simulink model "RFID"  (R2023a)
settings: Solver=VariableStepAuto  StartTime=0.0  StopTime=10.0  RelTol=1e-3
(part 2 of 2)

== system RFID/Profinet_network ==
  Bus Element In2 : Inport  PortName=IOLink_master_Profinet_serial_data_profinet
  Bus Element In1 : Inport  Port=2  PortName="XGSZ84 PNT  _serial_data_Profinet"
  Bus Element In3 : Inport  Port=3  PortName=XGCS 850C 201_Profinet_Data
  Bus Element Out1 : Outport  PortName=Profinet_Sensor_fieldbus

== system RFID/RFID_CANJ ==
  XGCS460B201 : Subsystem
      settings: PortSchema="{\"entries\":[{\"content\":{\"headerSize\":26,\"margin\":15,\"minimumSpacing\":25,\"sides\":[{\"content\":{},\"type\":\"ConnectorPlacement.EquallySpacedRectSide\",\"uuid\":\"ff8f3bf2-d6f6-4ecc-9677-a0e5f5ade440\"},{\"content\":{\"connectorIds\":[\"Out1\"],\"side\":\"RIGHT\"},\"type\":\"ConnectorPlacement.EquallySpacedRectSide\",\"uuid\":\"fe155757-f3d5-40d8-a583-dbbc24843437\"},{\"content\":{\"side\":\"TOP\"},\"type\":\"ConnectorPlacement.EquallySpacedRectSide\",\"uuid\":\"51bc4fd0-0675-45de-93bd-0dc8d94c5489\"}]},\"type\":\"ConnectorPlacement.EquallySpacedConnector\",\"uuid\":\"7eb8fdf8-dbe2-49f3-b9bd-384f85dcc997\"}],\"packageUris\":[\"http://schema.mathworks.com/mf0/Connector/R2020b\"],\"version\":\"1.0\"}"
  XGCS460B202_CANJ_Data1 : Outport  PortName=XGCS460B201_CANJ_Data
  wires:
  XGCS460B201/1(XGCS460B201_CANJ_Data) -> XGCS460B202_CANJ_Data1/1

== system RFID/RFID_EthernetIP ==
  "XGCS 850C 201 " : Subsystem
      settings: PortSchema="{\"entries\":[{\"content\":{\"headerSize\":26,\"margin\":15,\"minimumSpacing\":25,\"sides\":[{\"content\":{},\"type\":\"ConnectorPlacement.EquallySpacedRectSide\",\"uuid\":\"ff8f3bf2-d6f6-4ecc-9677-a0e5f5ade440\"},{\"content\":{\"side\":\"RIGHT\"},\"type\":\"ConnectorPlacement.EquallySpacedRectSide\",\"uuid\":\"fe155757-f3d5-40d8-a583-dbbc24843437\"},{\"content\":{\"connectorIds\":[\"Out1\"],\"side\":\"TOP\"},\"type\":\"ConnectorPlacement.EquallySpacedRectSide\",\"uuid\":\"51bc4fd0-0675-45de-93bd-0dc8d94c5489\"}]},\"type\":\"ConnectorPlacement.EquallySpacedConnector\",\"uuid\":\"7eb8fdf8-dbe2-49f3-b9bd-384f85dcc997\"}],\"packageUris\":[\"http://schema.mathworks.com/mf0/Connector/R2020b\"],\"version\":\"1.0\"}"
  XGCS 850C 201_Ethernetp_Data1 : Outport  PortName=XGCS 850C 201_Ethernetp_Data
  wires:
  "XGCS 850C 201 "/1(XGCS 850C 201_Ethernetp_Data) -> XGCS 850C 201_Ethernetp_Data1/1

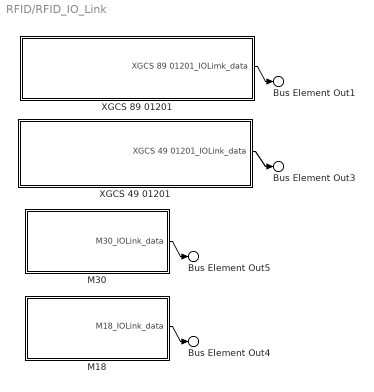
== system RFID/RFID_IO_Link ==
  M18 : Subsystem
      settings: PortSchema="{\"entries\":[{\"content\":{\"headerSize\":26,\"margin\":15,\"minimumSpacing\":25,\"sides\":[{\"content\":{},\"type\":\"ConnectorPlacement.EquallySpacedRectSide\",\"uuid\":\"ff8f3bf2-d6f6-4ecc-9677-a0e5f5ade440\"},{\"content\":{\"connectorIds\":[\"Out1\"],\"side\":\"RIGHT\"},\"type\":\"ConnectorPlacement.EquallySpacedRectSide\",\"uuid\":\"fe155757-f3d5-40d8-a583-dbbc24843437\"},{\"content\":{\"side\":\"TOP\"},\"type\":\"ConnectorPlacement.EquallySpacedRectSide\",\"uuid\":\"51bc4fd0-0675-45de-93bd-0dc8d94c5489\"}]},\"type\":\"ConnectorPlacement.EquallySpacedConnector\",\"uuid\":\"7eb8fdf8-dbe2-49f3-b9bd-384f85dcc997\"}],\"packageUris\":[\"http://schema.mathworks.com/mf0/Connector/R2020b\"],\"version\":\"1.0\"}"
  M30 : Subsystem
      settings: PortSchema="{\"entries\":[{\"content\":{\"headerSize\":26,\"margin\":15,\"minimumSpacing\":25,\"sides\":[{\"content\":{},\"type\":\"ConnectorPlacement.EquallySpacedRectSide\",\"uuid\":\"ff8f3bf2-d6f6-4ecc-9677-a0e5f5ade440\"},{\"content\":{\"connectorIds\":[\"Out1\"],\"side\":\"RIGHT\"},\"type\":\"ConnectorPlacement.EquallySpacedRectSide\",\"uuid\":\"fe155757-f3d5-40d8-a583-dbbc24843437\"},{\"content\":{\"side\":\"TOP\"},\"type\":\"ConnectorPlacement.EquallySpacedRectSide\",\"uuid\":\"51bc4fd0-0675-45de-93bd-0dc8d94c5489\"}]},\"type\":\"ConnectorPlacement.EquallySpacedConnector\",\"uuid\":\"7eb8fdf8-dbe2-49f3-b9bd-384f85dcc997\"}],\"packageUris\":[\"http://schema.mathworks.com/mf0/Connector/R2020b\"],\"version\":\"1.0\"}"
  XGCS 49 01201 : Subsystem
      settings: PortSchema="{\"entries\":[{\"content\":{\"headerSize\":26,\"margin\":15,\"minimumSpacing\":25,\"sides\":[{\"content\":{},\"type\":\"ConnectorPlacement.EquallySpacedRectSide\",\"uuid\":\"ff8f3bf2-d6f6-4ecc-9677-a0e5f5ade440\"},{\"content\":{\"connectorIds\":[\"Out1\"],\"side\":\"RIGHT\"},\"type\":\"ConnectorPlacement.EquallySpacedRectSide\",\"uuid\":\"fe155757-f3d5-40d8-a583-dbbc24843437\"},{\"content\":{\"side\":\"TOP\"},\"type\":\"ConnectorPlacement.EquallySpacedRectSide\",\"uuid\":\"51bc4fd0-0675-45de-93bd-0dc8d94c5489\"}]},\"type\":\"ConnectorPlacement.EquallySpacedConnector\",\"uuid\":\"7eb8fdf8-dbe2-49f3-b9bd-384f85dcc997\"}],\"packageUris\":[\"http://schema.mathworks.com/mf0/Connector/R2020b\"],\"version\":\"1.0\"}"
  XGCS 89 01201 : Subsystem
      settings: PortSchema="{\"entries\":[{\"content\":{\"headerSize\":26,\"margin\":15,\"minimumSpacing\":25,\"sides\":[{\"content\":{},\"type\":\"ConnectorPlacement.EquallySpacedRectSide\",\"uuid\":\"ff8f3bf2-d6f6-4ecc-9677-a0e5f5ade440\"},{\"content\":{\"connectorIds\":[\"Out1\"],\"side\":\"RIGHT\"},\"type\":\"ConnectorPlacement.EquallySpacedRectSide\",\"uuid\":\"fe155757-f3d5-40d8-a583-dbbc24843437\"},{\"content\":{\"side\":\"TOP\"},\"type\":\"ConnectorPlacement.EquallySpacedRectSide\",\"uuid\":\"51bc4fd0-0675-45de-93bd-0dc8d94c5489\"}]},\"type\":\"ConnectorPlacement.EquallySpacedConnector\",\"uuid\":\"7eb8fdf8-dbe2-49f3-b9bd-384f85dcc997\"}],\"packageUris\":[\"http://schema.mathworks.com/mf0/Connector/R2020b\"],\"version\":\"1.0\"}"
  Bus Element Out1 : Outport  PortName=XGCS 89 01201_IOLimk_data
  Bus Element Out3 : Outport  Port=2  PortName=XGCS 49 01201_IOLink_data
  Bus Element Out4 : Outport  Port=3  PortName=M18_IOLink_data
  Bus Element Out5 : Outport  Port=4  PortName=M30_IOLink_data
  wires:
  XGCS 89 01201/1(XGCS 89 01201_IOLimk_data) -> Bus Element Out1/1
  XGCS 49 01201/1(XGCS 49 01201_IOLink_data) -> Bus Element Out3/1
  M30/1(M30_IOLink_data) -> Bus Element Out5/1
  M18/1(M18_IOLink_data) -> Bus Element Out4/1

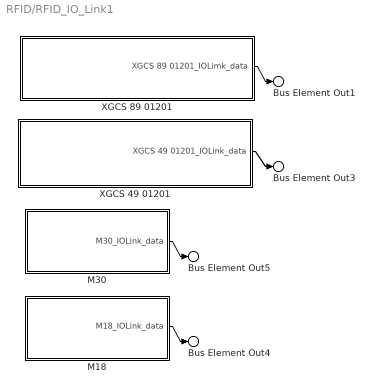
== system RFID/RFID_IO_Link1 ==
  M18 : Subsystem
      settings: PortSchema="{\"entries\":[{\"content\":{\"headerSize\":26,\"margin\":15,\"minimumSpacing\":25,\"sides\":[{\"content\":{},\"type\":\"ConnectorPlacement.EquallySpacedRectSide\",\"uuid\":\"ff8f3bf2-d6f6-4ecc-9677-a0e5f5ade440\"},{\"content\":{\"connectorIds\":[\"Out1\"],\"side\":\"RIGHT\"},\"type\":\"ConnectorPlacement.EquallySpacedRectSide\",\"uuid\":\"fe155757-f3d5-40d8-a583-dbbc24843437\"},{\"content\":{\"side\":\"TOP\"},\"type\":\"ConnectorPlacement.EquallySpacedRectSide\",\"uuid\":\"51bc4fd0-0675-45de-93bd-0dc8d94c5489\"}]},\"type\":\"ConnectorPlacement.EquallySpacedConnector\",\"uuid\":\"7eb8fdf8-dbe2-49f3-b9bd-384f85dcc997\"}],\"packageUris\":[\"http://schema.mathworks.com/mf0/Connector/R2020b\"],\"version\":\"1.0\"}"
  M30 : Subsystem
      settings: PortSchema="{\"entries\":[{\"content\":{\"headerSize\":26,\"margin\":15,\"minimumSpacing\":25,\"sides\":[{\"content\":{},\"type\":\"ConnectorPlacement.EquallySpacedRectSide\",\"uuid\":\"ff8f3bf2-d6f6-4ecc-9677-a0e5f5ade440\"},{\"content\":{\"connectorIds\":[\"Out1\"],\"side\":\"RIGHT\"},\"type\":\"ConnectorPlacement.EquallySpacedRectSide\",\"uuid\":\"fe155757-f3d5-40d8-a583-dbbc24843437\"},{\"content\":{\"side\":\"TOP\"},\"type\":\"ConnectorPlacement.EquallySpacedRectSide\",\"uuid\":\"51bc4fd0-0675-45de-93bd-0dc8d94c5489\"}]},\"type\":\"ConnectorPlacement.EquallySpacedConnector\",\"uuid\":\"7eb8fdf8-dbe2-49f3-b9bd-384f85dcc997\"}],\"packageUris\":[\"http://schema.mathworks.com/mf0/Connector/R2020b\"],\"version\":\"1.0\"}"
  XGCS 49 01201 : Subsystem
      settings: PortSchema="{\"entries\":[{\"content\":{\"headerSize\":26,\"margin\":15,\"minimumSpacing\":25,\"sides\":[{\"content\":{},\"type\":\"ConnectorPlacement.EquallySpacedRectSide\",\"uuid\":\"ff8f3bf2-d6f6-4ecc-9677-a0e5f5ade440\"},{\"content\":{\"connectorIds\":[\"Out1\"],\"side\":\"RIGHT\"},\"type\":\"ConnectorPlacement.EquallySpacedRectSide\",\"uuid\":\"fe155757-f3d5-40d8-a583-dbbc24843437\"},{\"content\":{\"side\":\"TOP\"},\"type\":\"ConnectorPlacement.EquallySpacedRectSide\",\"uuid\":\"51bc4fd0-0675-45de-93bd-0dc8d94c5489\"}]},\"type\":\"ConnectorPlacement.EquallySpacedConnector\",\"uuid\":\"7eb8fdf8-dbe2-49f3-b9bd-384f85dcc997\"}],\"packageUris\":[\"http://schema.mathworks.com/mf0/Connector/R2020b\"],\"version\":\"1.0\"}"
  XGCS 89 01201 : Subsystem
      settings: PortSchema="{\"entries\":[{\"content\":{\"headerSize\":26,\"margin\":15,\"minimumSpacing\":25,\"sides\":[{\"content\":{},\"type\":\"ConnectorPlacement.EquallySpacedRectSide\",\"uuid\":\"ff8f3bf2-d6f6-4ecc-9677-a0e5f5ade440\"},{\"content\":{\"connectorIds\":[\"Out1\"],\"side\":\"RIGHT\"},\"type\":\"ConnectorPlacement.EquallySpacedRectSide\",\"uuid\":\"fe155757-f3d5-40d8-a583-dbbc24843437\"},{\"content\":{\"side\":\"TOP\"},\"type\":\"ConnectorPlacement.EquallySpacedRectSide\",\"uuid\":\"51bc4fd0-0675-45de-93bd-0dc8d94c5489\"}]},\"type\":\"ConnectorPlacement.EquallySpacedConnector\",\"uuid\":\"7eb8fdf8-dbe2-49f3-b9bd-384f85dcc997\"}],\"packageUris\":[\"http://schema.mathworks.com/mf0/Connector/R2020b\"],\"version\":\"1.0\"}"
  Bus Element Out1 : Outport  PortName=XGCS 89 01201_IOLimk_data
  Bus Element Out3 : Outport  Port=2  PortName=XGCS 49 01201_IOLink_data
  Bus Element Out4 : Outport  Port=3  PortName=M18_IOLink_data
  Bus Element Out5 : Outport  Port=4  PortName=M30_IOLink_data
  wires:
  XGCS 89 01201/1(XGCS 89 01201_IOLimk_data) -> Bus Element Out1/1
  XGCS 49 01201/1(XGCS 49 01201_IOLink_data) -> Bus Element Out3/1
  M30/1(M30_IOLink_data) -> Bus Element Out5/1
  M18/1(M18_IOLink_data) -> Bus Element Out4/1

== system RFID/RFID_Modbus ==
  XGCS 850C 201 : Subsystem
      settings: PortSchema="{\"entries\":[{\"content\":{\"headerSize\":26,\"margin\":15,\"minimumSpacing\":25,\"sides\":[{\"content\":{},\"type\":\"ConnectorPlacement.EquallySpacedRectSide\",\"uuid\":\"ff8f3bf2-d6f6-4ecc-9677-a0e5f5ade440\"},{\"content\":{\"side\":\"RIGHT\"},\"type\":\"ConnectorPlacement.EquallySpacedRectSide\",\"uuid\":\"fe155757-f3d5-40d8-a583-dbbc24843437\"},{\"content\":{\"connectorIds\":[\"Out1\"],\"side\":\"TOP\"},\"type\":\"ConnectorPlacement.EquallySpacedRectSide\",\"uuid\":\"51bc4fd0-0675-45de-93bd-0dc8d94c5489\"}]},\"type\":\"ConnectorPlacement.EquallySpacedConnector\",\"uuid\":\"7eb8fdf8-dbe2-49f3-b9bd-384f85dcc997\"}],\"packageUris\":[\"http://schema.mathworks.com/mf0/Connector/R2020b\"],\"version\":\"1.0\"}"
  XGCS 850C 201_ModusTCp_Data1 : Outport  PortName=XGCS 850C 201_ModusTCp_Data
  wires:
  XGCS 850C 201/1(XGCS 850C 201_ModusTCp_Data) -> XGCS 850C 201_ModusTCp_Data1/1

== system RFID/RFID_PNP ==
  "XGCS49 1 B201 " : Subsystem
      settings: PortSchema="{\"entries\":[{\"content\":{\"headerSize\":26,\"margin\":15,\"minimumSpacing\":25,\"sides\":[{\"content\":{},\"type\":\"ConnectorPlacement.EquallySpacedRectSide\",\"uuid\":\"ff8f3bf2-d6f6-4ecc-9677-a0e5f5ade440\"},{\"content\":{\"connectorIds\":[\"Out1\"],\"side\":\"RIGHT\"},\"type\":\"ConnectorPlacement.EquallySpacedRectSide\",\"uuid\":\"fe155757-f3d5-40d8-a583-dbbc24843437\"},{\"content\":{\"side\":\"TOP\"},\"type\":\"ConnectorPlacement.EquallySpacedRectSide\",\"uuid\":\"51bc4fd0-0675-45de-93bd-0dc8d94c5489\"}]},\"type\":\"ConnectorPlacement.EquallySpacedConnector\",\"uuid\":\"7eb8fdf8-dbe2-49f3-b9bd-384f85dcc997\"}],\"packageUris\":[\"http://schema.mathworks.com/mf0/Connector/R2020b\"],\"version\":\"1.0\"}"
  XGCS49 1 B201_PNP_Data1 : Outport  PortName=XGCS49 1 B201_PNP_Data
  wires:
  "XGCS49 1 B201 "/1(XGCS49 1 B201_PNP_Data) -> XGCS49 1 B201_PNP_Data1/1

== system RFID/RFID_Profinet ==
  "XGCS 850C 201 " : Subsystem
      settings: PortSchema="{\"entries\":[{\"content\":{\"headerSize\":26,\"margin\":15,\"minimumSpacing\":25,\"sides\":[{\"content\":{},\"type\":\"ConnectorPlacement.EquallySpacedRectSide\",\"uuid\":\"ff8f3bf2-d6f6-4ecc-9677-a0e5f5ade440\"},{\"content\":{\"side\":\"RIGHT\"},\"type\":\"ConnectorPlacement.EquallySpacedRectSide\",\"uuid\":\"fe155757-f3d5-40d8-a583-dbbc24843437\"},{\"content\":{\"connectorIds\":[\"Out1\"],\"side\":\"TOP\"},\"type\":\"ConnectorPlacement.EquallySpacedRectSide\",\"uuid\":\"51bc4fd0-0675-45de-93bd-0dc8d94c5489\"}]},\"type\":\"ConnectorPlacement.EquallySpacedConnector\",\"uuid\":\"7eb8fdf8-dbe2-49f3-b9bd-384f85dcc997\"}],\"packageUris\":[\"http://schema.mathworks.com/mf0/Connector/R2020b\"],\"version\":\"1.0\"}"
  Bus Element Out1 : Outport  PortName=XGCS 850C 201_Profinet_Data
  wires:
  "XGCS 850C 201 "/1(XGCS 850C 201_Profinet_Data) -> Bus Element Out1/1

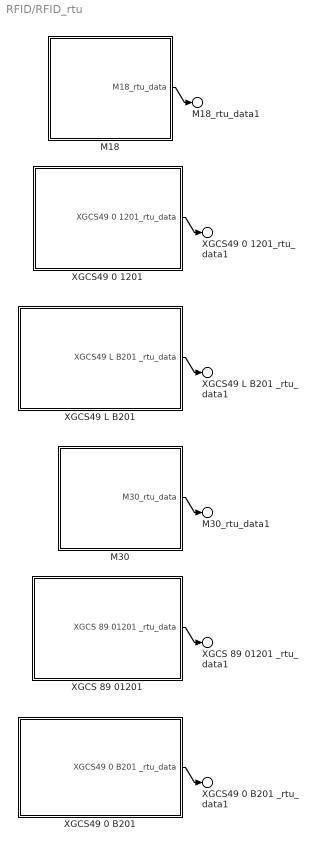
== system RFID/RFID_rtu ==
  M18 : Subsystem
      settings: PortSchema="{\"entries\":[{\"content\":{\"headerSize\":26,\"margin\":15,\"minimumSpacing\":25,\"sides\":[{\"content\":{},\"type\":\"ConnectorPlacement.EquallySpacedRectSide\",\"uuid\":\"ff8f3bf2-d6f6-4ecc-9677-a0e5f5ade440\"},{\"content\":{\"connectorIds\":[\"Out1\"],\"side\":\"RIGHT\"},\"type\":\"ConnectorPlacement.EquallySpacedRectSide\",\"uuid\":\"fe155757-f3d5-40d8-a583-dbbc24843437\"},{\"content\":{\"side\":\"TOP\"},\"type\":\"ConnectorPlacement.EquallySpacedRectSide\",\"uuid\":\"51bc4fd0-0675-45de-93bd-0dc8d94c5489\"}]},\"type\":\"ConnectorPlacement.EquallySpacedConnector\",\"uuid\":\"7eb8fdf8-dbe2-49f3-b9bd-384f85dcc997\"}],\"packageUris\":[\"http://schema.mathworks.com/mf0/Connector/R2020b\"],\"version\":\"1.0\"}"
  M30 : Subsystem
      settings: PortSchema="{\"entries\":[{\"content\":{\"headerSize\":26,\"margin\":15,\"minimumSpacing\":25,\"sides\":[{\"content\":{},\"type\":\"ConnectorPlacement.EquallySpacedRectSide\",\"uuid\":\"ff8f3bf2-d6f6-4ecc-9677-a0e5f5ade440\"},{\"content\":{\"connectorIds\":[\"Out1\"],\"side\":\"RIGHT\"},\"type\":\"ConnectorPlacement.EquallySpacedRectSide\",\"uuid\":\"fe155757-f3d5-40d8-a583-dbbc24843437\"},{\"content\":{\"side\":\"TOP\"},\"type\":\"ConnectorPlacement.EquallySpacedRectSide\",\"uuid\":\"51bc4fd0-0675-45de-93bd-0dc8d94c5489\"}]},\"type\":\"ConnectorPlacement.EquallySpacedConnector\",\"uuid\":\"7eb8fdf8-dbe2-49f3-b9bd-384f85dcc997\"}],\"packageUris\":[\"http://schema.mathworks.com/mf0/Connector/R2020b\"],\"version\":\"1.0\"}"
  "XGCS 89 01201 " : Subsystem
      settings: PortSchema="{\"entries\":[{\"content\":{\"headerSize\":26,\"margin\":15,\"minimumSpacing\":25,\"sides\":[{\"content\":{},\"type\":\"ConnectorPlacement.EquallySpacedRectSide\",\"uuid\":\"ff8f3bf2-d6f6-4ecc-9677-a0e5f5ade440\"},{\"content\":{\"connectorIds\":[\"Out1\"],\"side\":\"RIGHT\"},\"type\":\"ConnectorPlacement.EquallySpacedRectSide\",\"uuid\":\"fe155757-f3d5-40d8-a583-dbbc24843437\"},{\"content\":{\"side\":\"TOP\"},\"type\":\"ConnectorPlacement.EquallySpacedRectSide\",\"uuid\":\"51bc4fd0-0675-45de-93bd-0dc8d94c5489\"}]},\"type\":\"ConnectorPlacement.EquallySpacedConnector\",\"uuid\":\"7eb8fdf8-dbe2-49f3-b9bd-384f85dcc997\"}],\"packageUris\":[\"http://schema.mathworks.com/mf0/Connector/R2020b\"],\"version\":\"1.0\"}"
  "XGCS49 0 1201 " : Subsystem
      settings: PortSchema="{\"entries\":[{\"content\":{\"headerSize\":26,\"margin\":15,\"minimumSpacing\":25,\"sides\":[{\"content\":{},\"type\":\"ConnectorPlacement.EquallySpacedRectSide\",\"uuid\":\"ff8f3bf2-d6f6-4ecc-9677-a0e5f5ade440\"},{\"content\":{\"connectorIds\":[\"Out1\"],\"side\":\"RIGHT\"},\"type\":\"ConnectorPlacement.EquallySpacedRectSide\",\"uuid\":\"fe155757-f3d5-40d8-a583-dbbc24843437\"},{\"content\":{\"side\":\"TOP\"},\"type\":\"ConnectorPlacement.EquallySpacedRectSide\",\"uuid\":\"51bc4fd0-0675-45de-93bd-0dc8d94c5489\"}]},\"type\":\"ConnectorPlacement.EquallySpacedConnector\",\"uuid\":\"7eb8fdf8-dbe2-49f3-b9bd-384f85dcc997\"}],\"packageUris\":[\"http://schema.mathworks.com/mf0/Connector/R2020b\"],\"version\":\"1.0\"}"
  "XGCS49 0 B201 " : Subsystem
      settings: PortSchema="{\"entries\":[{\"content\":{\"headerSize\":26,\"margin\":15,\"minimumSpacing\":25,\"sides\":[{\"content\":{},\"type\":\"ConnectorPlacement.EquallySpacedRectSide\",\"uuid\":\"ff8f3bf2-d6f6-4ecc-9677-a0e5f5ade440\"},{\"content\":{\"connectorIds\":[\"Out1\"],\"side\":\"RIGHT\"},\"type\":\"ConnectorPlacement.EquallySpacedRectSide\",\"uuid\":\"fe155757-f3d5-40d8-a583-dbbc24843437\"},{\"content\":{\"side\":\"TOP\"},\"type\":\"ConnectorPlacement.EquallySpacedRectSide\",\"uuid\":\"51bc4fd0-0675-45de-93bd-0dc8d94c5489\"}]},\"type\":\"ConnectorPlacement.EquallySpacedConnector\",\"uuid\":\"7eb8fdf8-dbe2-49f3-b9bd-384f85dcc997\"}],\"packageUris\":[\"http://schema.mathworks.com/mf0/Connector/R2020b\"],\"version\":\"1.0\"}"
  "XGCS49 L B201 " : Subsystem
      settings: PortSchema="{\"entries\":[{\"content\":{\"headerSize\":26,\"margin\":15,\"minimumSpacing\":25,\"sides\":[{\"content\":{},\"type\":\"ConnectorPlacement.EquallySpacedRectSide\",\"uuid\":\"ff8f3bf2-d6f6-4ecc-9677-a0e5f5ade440\"},{\"content\":{\"connectorIds\":[\"Out1\"],\"side\":\"RIGHT\"},\"type\":\"ConnectorPlacement.EquallySpacedRectSide\",\"uuid\":\"fe155757-f3d5-40d8-a583-dbbc24843437\"},{\"content\":{\"side\":\"TOP\"},\"type\":\"ConnectorPlacement.EquallySpacedRectSide\",\"uuid\":\"51bc4fd0-0675-45de-93bd-0dc8d94c5489\"}]},\"type\":\"ConnectorPlacement.EquallySpacedConnector\",\"uuid\":\"7eb8fdf8-dbe2-49f3-b9bd-384f85dcc997\"}],\"packageUris\":[\"http://schema.mathworks.com/mf0/Connector/R2020b\"],\"version\":\"1.0\"}"
  M18_rtu_data1 : Outport  PortName=M18_rtu_data
  M30_rtu_data1 : Outport  Port=2  PortName=M30_rtu_data
  XGCS49 0 1201_rtu_data1 : Outport  Port=3  PortName=XGCS49 0 1201_rtu_data
  XGCS 89 01201 _rtu_data1 : Outport  Port=4  PortName=XGCS 89 01201 _rtu_data
  XGCS49 0 B201 _rtu_data1 : Outport  Port=5  PortName=XGCS49 0 B201 _rtu_data
  XGCS49 L B201 _rtu_data1 : Outport  Port=6  PortName=XGCS49 L B201 _rtu_data
  wires:
  "XGCS 89 01201 "/1(XGCS 89 01201 _rtu_data) -> XGCS 89 01201 _rtu_data1/1
  "XGCS49 L B201 "/1(XGCS49 L B201 _rtu_data) -> XGCS49 L B201 _rtu_data1/1
  "XGCS49 0 B201 "/1(XGCS49 0 B201 _rtu_data) -> XGCS49 0 B201 _rtu_data1/1
  M18/1(M18_rtu_data) -> M18_rtu_data1/1
  M30/1(M30_rtu_data) -> M30_rtu_data1/1
  "XGCS49 0 1201 "/1(XGCS49 0 1201_rtu_data) -> XGCS49 0 1201_rtu_data1/1

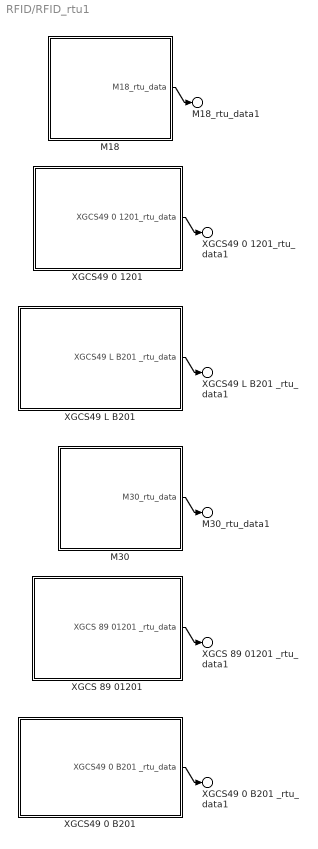
== system RFID/RFID_rtu1 ==
  M18 : Subsystem
      settings: PortSchema="{\"entries\":[{\"content\":{\"headerSize\":26,\"margin\":15,\"minimumSpacing\":25,\"sides\":[{\"content\":{},\"type\":\"ConnectorPlacement.EquallySpacedRectSide\",\"uuid\":\"ff8f3bf2-d6f6-4ecc-9677-a0e5f5ade440\"},{\"content\":{\"connectorIds\":[\"Out1\"],\"side\":\"RIGHT\"},\"type\":\"ConnectorPlacement.EquallySpacedRectSide\",\"uuid\":\"fe155757-f3d5-40d8-a583-dbbc24843437\"},{\"content\":{\"side\":\"TOP\"},\"type\":\"ConnectorPlacement.EquallySpacedRectSide\",\"uuid\":\"51bc4fd0-0675-45de-93bd-0dc8d94c5489\"}]},\"type\":\"ConnectorPlacement.EquallySpacedConnector\",\"uuid\":\"7eb8fdf8-dbe2-49f3-b9bd-384f85dcc997\"}],\"packageUris\":[\"http://schema.mathworks.com/mf0/Connector/R2020b\"],\"version\":\"1.0\"}"
  M30 : Subsystem
      settings: PortSchema="{\"entries\":[{\"content\":{\"headerSize\":26,\"margin\":15,\"minimumSpacing\":25,\"sides\":[{\"content\":{},\"type\":\"ConnectorPlacement.EquallySpacedRectSide\",\"uuid\":\"ff8f3bf2-d6f6-4ecc-9677-a0e5f5ade440\"},{\"content\":{\"connectorIds\":[\"Out1\"],\"side\":\"RIGHT\"},\"type\":\"ConnectorPlacement.EquallySpacedRectSide\",\"uuid\":\"fe155757-f3d5-40d8-a583-dbbc24843437\"},{\"content\":{\"side\":\"TOP\"},\"type\":\"ConnectorPlacement.EquallySpacedRectSide\",\"uuid\":\"51bc4fd0-0675-45de-93bd-0dc8d94c5489\"}]},\"type\":\"ConnectorPlacement.EquallySpacedConnector\",\"uuid\":\"7eb8fdf8-dbe2-49f3-b9bd-384f85dcc997\"}],\"packageUris\":[\"http://schema.mathworks.com/mf0/Connector/R2020b\"],\"version\":\"1.0\"}"
  "XGCS 89 01201 " : Subsystem
      settings: PortSchema="{\"entries\":[{\"content\":{\"headerSize\":26,\"margin\":15,\"minimumSpacing\":25,\"sides\":[{\"content\":{},\"type\":\"ConnectorPlacement.EquallySpacedRectSide\",\"uuid\":\"ff8f3bf2-d6f6-4ecc-9677-a0e5f5ade440\"},{\"content\":{\"connectorIds\":[\"Out1\"],\"side\":\"RIGHT\"},\"type\":\"ConnectorPlacement.EquallySpacedRectSide\",\"uuid\":\"fe155757-f3d5-40d8-a583-dbbc24843437\"},{\"content\":{\"side\":\"TOP\"},\"type\":\"ConnectorPlacement.EquallySpacedRectSide\",\"uuid\":\"51bc4fd0-0675-45de-93bd-0dc8d94c5489\"}]},\"type\":\"ConnectorPlacement.EquallySpacedConnector\",\"uuid\":\"7eb8fdf8-dbe2-49f3-b9bd-384f85dcc997\"}],\"packageUris\":[\"http://schema.mathworks.com/mf0/Connector/R2020b\"],\"version\":\"1.0\"}"
  "XGCS49 0 1201 " : Subsystem
      settings: PortSchema="{\"entries\":[{\"content\":{\"headerSize\":26,\"margin\":15,\"minimumSpacing\":25,\"sides\":[{\"content\":{},\"type\":\"ConnectorPlacement.EquallySpacedRectSide\",\"uuid\":\"ff8f3bf2-d6f6-4ecc-9677-a0e5f5ade440\"},{\"content\":{\"connectorIds\":[\"Out1\"],\"side\":\"RIGHT\"},\"type\":\"ConnectorPlacement.EquallySpacedRectSide\",\"uuid\":\"fe155757-f3d5-40d8-a583-dbbc24843437\"},{\"content\":{\"side\":\"TOP\"},\"type\":\"ConnectorPlacement.EquallySpacedRectSide\",\"uuid\":\"51bc4fd0-0675-45de-93bd-0dc8d94c5489\"}]},\"type\":\"ConnectorPlacement.EquallySpacedConnector\",\"uuid\":\"7eb8fdf8-dbe2-49f3-b9bd-384f85dcc997\"}],\"packageUris\":[\"http://schema.mathworks.com/mf0/Connector/R2020b\"],\"version\":\"1.0\"}"
  "XGCS49 0 B201 " : Subsystem
      settings: PortSchema="{\"entries\":[{\"content\":{\"headerSize\":26,\"margin\":15,\"minimumSpacing\":25,\"sides\":[{\"content\":{},\"type\":\"ConnectorPlacement.EquallySpacedRectSide\",\"uuid\":\"ff8f3bf2-d6f6-4ecc-9677-a0e5f5ade440\"},{\"content\":{\"connectorIds\":[\"Out1\"],\"side\":\"RIGHT\"},\"type\":\"ConnectorPlacement.EquallySpacedRectSide\",\"uuid\":\"fe155757-f3d5-40d8-a583-dbbc24843437\"},{\"content\":{\"side\":\"TOP\"},\"type\":\"ConnectorPlacement.EquallySpacedRectSide\",\"uuid\":\"51bc4fd0-0675-45de-93bd-0dc8d94c5489\"}]},\"type\":\"ConnectorPlacement.EquallySpacedConnector\",\"uuid\":\"7eb8fdf8-dbe2-49f3-b9bd-384f85dcc997\"}],\"packageUris\":[\"http://schema.mathworks.com/mf0/Connector/R2020b\"],\"version\":\"1.0\"}"
  "XGCS49 L B201 " : Subsystem
      settings: PortSchema="{\"entries\":[{\"content\":{\"headerSize\":26,\"margin\":15,\"minimumSpacing\":25,\"sides\":[{\"content\":{},\"type\":\"ConnectorPlacement.EquallySpacedRectSide\",\"uuid\":\"ff8f3bf2-d6f6-4ecc-9677-a0e5f5ade440\"},{\"content\":{\"connectorIds\":[\"Out1\"],\"side\":\"RIGHT\"},\"type\":\"ConnectorPlacement.EquallySpacedRectSide\",\"uuid\":\"fe155757-f3d5-40d8-a583-dbbc24843437\"},{\"content\":{\"side\":\"TOP\"},\"type\":\"ConnectorPlacement.EquallySpacedRectSide\",\"uuid\":\"51bc4fd0-0675-45de-93bd-0dc8d94c5489\"}]},\"type\":\"ConnectorPlacement.EquallySpacedConnector\",\"uuid\":\"7eb8fdf8-dbe2-49f3-b9bd-384f85dcc997\"}],\"packageUris\":[\"http://schema.mathworks.com/mf0/Connector/R2020b\"],\"version\":\"1.0\"}"
  M18_rtu_data1 : Outport  PortName=M18_rtu_data
  M30_rtu_data1 : Outport  Port=2  PortName=M30_rtu_data
  XGCS49 0 1201_rtu_data1 : Outport  Port=3  PortName=XGCS49 0 1201_rtu_data
  XGCS 89 01201 _rtu_data1 : Outport  Port=4  PortName=XGCS 89 01201 _rtu_data
  XGCS49 0 B201 _rtu_data1 : Outport  Port=5  PortName=XGCS49 0 B201 _rtu_data
  XGCS49 L B201 _rtu_data1 : Outport  Port=6  PortName=XGCS49 L B201 _rtu_data
  wires:
  "XGCS 89 01201 "/1(XGCS 89 01201 _rtu_data) -> XGCS 89 01201 _rtu_data1/1
  "XGCS49 L B201 "/1(XGCS49 L B201 _rtu_data) -> XGCS49 L B201 _rtu_data1/1
  "XGCS49 0 B201 "/1(XGCS49 0 B201 _rtu_data) -> XGCS49 0 B201 _rtu_data1/1
  M18/1(M18_rtu_data) -> M18_rtu_data1/1
  M30/1(M30_rtu_data) -> M30_rtu_data1/1
  "XGCS49 0 1201 "/1(XGCS49 0 1201_rtu_data) -> XGCS49 0 1201_rtu_data1/1

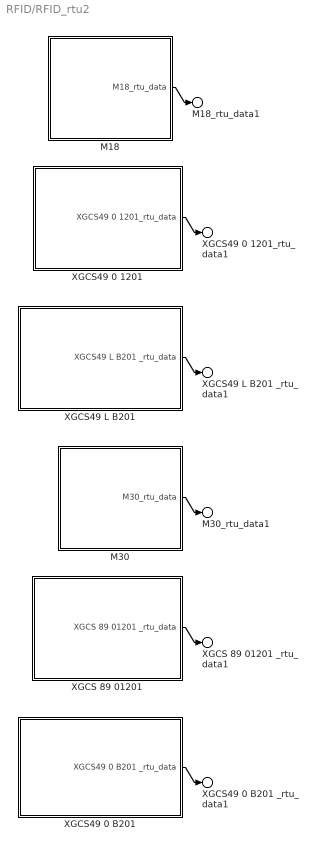
== system RFID/RFID_rtu2 ==
  M18 : Subsystem
      settings: PortSchema="{\"entries\":[{\"content\":{\"headerSize\":26,\"margin\":15,\"minimumSpacing\":25,\"sides\":[{\"content\":{},\"type\":\"ConnectorPlacement.EquallySpacedRectSide\",\"uuid\":\"ff8f3bf2-d6f6-4ecc-9677-a0e5f5ade440\"},{\"content\":{\"connectorIds\":[\"Out1\"],\"side\":\"RIGHT\"},\"type\":\"ConnectorPlacement.EquallySpacedRectSide\",\"uuid\":\"fe155757-f3d5-40d8-a583-dbbc24843437\"},{\"content\":{\"side\":\"TOP\"},\"type\":\"ConnectorPlacement.EquallySpacedRectSide\",\"uuid\":\"51bc4fd0-0675-45de-93bd-0dc8d94c5489\"}]},\"type\":\"ConnectorPlacement.EquallySpacedConnector\",\"uuid\":\"7eb8fdf8-dbe2-49f3-b9bd-384f85dcc997\"}],\"packageUris\":[\"http://schema.mathworks.com/mf0/Connector/R2020b\"],\"version\":\"1.0\"}"
  M30 : Subsystem
      settings: PortSchema="{\"entries\":[{\"content\":{\"headerSize\":26,\"margin\":15,\"minimumSpacing\":25,\"sides\":[{\"content\":{},\"type\":\"ConnectorPlacement.EquallySpacedRectSide\",\"uuid\":\"ff8f3bf2-d6f6-4ecc-9677-a0e5f5ade440\"},{\"content\":{\"connectorIds\":[\"Out1\"],\"side\":\"RIGHT\"},\"type\":\"ConnectorPlacement.EquallySpacedRectSide\",\"uuid\":\"fe155757-f3d5-40d8-a583-dbbc24843437\"},{\"content\":{\"side\":\"TOP\"},\"type\":\"ConnectorPlacement.EquallySpacedRectSide\",\"uuid\":\"51bc4fd0-0675-45de-93bd-0dc8d94c5489\"}]},\"type\":\"ConnectorPlacement.EquallySpacedConnector\",\"uuid\":\"7eb8fdf8-dbe2-49f3-b9bd-384f85dcc997\"}],\"packageUris\":[\"http://schema.mathworks.com/mf0/Connector/R2020b\"],\"version\":\"1.0\"}"
  "XGCS 89 01201 " : Subsystem
      settings: PortSchema="{\"entries\":[{\"content\":{\"headerSize\":26,\"margin\":15,\"minimumSpacing\":25,\"sides\":[{\"content\":{},\"type\":\"ConnectorPlacement.EquallySpacedRectSide\",\"uuid\":\"ff8f3bf2-d6f6-4ecc-9677-a0e5f5ade440\"},{\"content\":{\"connectorIds\":[\"Out1\"],\"side\":\"RIGHT\"},\"type\":\"ConnectorPlacement.EquallySpacedRectSide\",\"uuid\":\"fe155757-f3d5-40d8-a583-dbbc24843437\"},{\"content\":{\"side\":\"TOP\"},\"type\":\"ConnectorPlacement.EquallySpacedRectSide\",\"uuid\":\"51bc4fd0-0675-45de-93bd-0dc8d94c5489\"}]},\"type\":\"ConnectorPlacement.EquallySpacedConnector\",\"uuid\":\"7eb8fdf8-dbe2-49f3-b9bd-384f85dcc997\"}],\"packageUris\":[\"http://schema.mathworks.com/mf0/Connector/R2020b\"],\"version\":\"1.0\"}"
  "XGCS49 0 1201 " : Subsystem
      settings: PortSchema="{\"entries\":[{\"content\":{\"headerSize\":26,\"margin\":15,\"minimumSpacing\":25,\"sides\":[{\"content\":{},\"type\":\"ConnectorPlacement.EquallySpacedRectSide\",\"uuid\":\"ff8f3bf2-d6f6-4ecc-9677-a0e5f5ade440\"},{\"content\":{\"connectorIds\":[\"Out1\"],\"side\":\"RIGHT\"},\"type\":\"ConnectorPlacement.EquallySpacedRectSide\",\"uuid\":\"fe155757-f3d5-40d8-a583-dbbc24843437\"},{\"content\":{\"side\":\"TOP\"},\"type\":\"ConnectorPlacement.EquallySpacedRectSide\",\"uuid\":\"51bc4fd0-0675-45de-93bd-0dc8d94c5489\"}]},\"type\":\"ConnectorPlacement.EquallySpacedConnector\",\"uuid\":\"7eb8fdf8-dbe2-49f3-b9bd-384f85dcc997\"}],\"packageUris\":[\"http://schema.mathworks.com/mf0/Connector/R2020b\"],\"version\":\"1.0\"}"
  "XGCS49 0 B201 " : Subsystem
      settings: PortSchema="{\"entries\":[{\"content\":{\"headerSize\":26,\"margin\":15,\"minimumSpacing\":25,\"sides\":[{\"content\":{},\"type\":\"ConnectorPlacement.EquallySpacedRectSide\",\"uuid\":\"ff8f3bf2-d6f6-4ecc-9677-a0e5f5ade440\"},{\"content\":{\"connectorIds\":[\"Out1\"],\"side\":\"RIGHT\"},\"type\":\"ConnectorPlacement.EquallySpacedRectSide\",\"uuid\":\"fe155757-f3d5-40d8-a583-dbbc24843437\"},{\"content\":{\"side\":\"TOP\"},\"type\":\"ConnectorPlacement.EquallySpacedRectSide\",\"uuid\":\"51bc4fd0-0675-45de-93bd-0dc8d94c5489\"}]},\"type\":\"ConnectorPlacement.EquallySpacedConnector\",\"uuid\":\"7eb8fdf8-dbe2-49f3-b9bd-384f85dcc997\"}],\"packageUris\":[\"http://schema.mathworks.com/mf0/Connector/R2020b\"],\"version\":\"1.0\"}"
  "XGCS49 L B201 " : Subsystem
      settings: PortSchema="{\"entries\":[{\"content\":{\"headerSize\":26,\"margin\":15,\"minimumSpacing\":25,\"sides\":[{\"content\":{},\"type\":\"ConnectorPlacement.EquallySpacedRectSide\",\"uuid\":\"ff8f3bf2-d6f6-4ecc-9677-a0e5f5ade440\"},{\"content\":{\"connectorIds\":[\"Out1\"],\"side\":\"RIGHT\"},\"type\":\"ConnectorPlacement.EquallySpacedRectSide\",\"uuid\":\"fe155757-f3d5-40d8-a583-dbbc24843437\"},{\"content\":{\"side\":\"TOP\"},\"type\":\"ConnectorPlacement.EquallySpacedRectSide\",\"uuid\":\"51bc4fd0-0675-45de-93bd-0dc8d94c5489\"}]},\"type\":\"ConnectorPlacement.EquallySpacedConnector\",\"uuid\":\"7eb8fdf8-dbe2-49f3-b9bd-384f85dcc997\"}],\"packageUris\":[\"http://schema.mathworks.com/mf0/Connector/R2020b\"],\"version\":\"1.0\"}"
  M18_rtu_data1 : Outport  PortName=M18_rtu_data
  M30_rtu_data1 : Outport  Port=2  PortName=M30_rtu_data
  XGCS49 0 1201_rtu_data1 : Outport  Port=3  PortName=XGCS49 0 1201_rtu_data
  XGCS 89 01201 _rtu_data1 : Outport  Port=4  PortName=XGCS 89 01201 _rtu_data
  XGCS49 0 B201 _rtu_data1 : Outport  Port=5  PortName=XGCS49 0 B201 _rtu_data
  XGCS49 L B201 _rtu_data1 : Outport  Port=6  PortName=XGCS49 L B201 _rtu_data
  wires:
  "XGCS 89 01201 "/1(XGCS 89 01201 _rtu_data) -> XGCS 89 01201 _rtu_data1/1
  "XGCS49 L B201 "/1(XGCS49 L B201 _rtu_data) -> XGCS49 L B201 _rtu_data1/1
  "XGCS49 0 B201 "/1(XGCS49 0 B201 _rtu_data) -> XGCS49 0 B201 _rtu_data1/1
  M18/1(M18_rtu_data) -> M18_rtu_data1/1
  M30/1(M30_rtu_data) -> M30_rtu_data1/1
  "XGCS49 0 1201 "/1(XGCS49 0 1201_rtu_data) -> XGCS49 0 1201_rtu_data1/1

== system RFID/TCSESU051F0 ==
  Bus Element In3 : Inport  PortName=IOLink_master_Profinet_serial_data_EthernetIP
  Bus Element In1 : Inport  Port=2  PortName=XGSZ 84 EIP _serial_data_ethernet
  Bus Element In2 : Inport  Port=3  PortName=XGCS 850C 201_Ethernetp_Data_2_swtich
  Bus Element Out1 : Outport  PortName=ethernet ip data

== system RFID/XGSZ 84 EIP  ==
  Bus Element In1 : Inport  PortName=M18_rtu_data_2_ethernet_box
  Bus Element In2 : Inport  Port=2  PortName=M30_rtu_data_2_ethernet_box
  Bus Element In3 : Inport  Port=3  PortName=XGCS49 0 1201_rtu_data_2_ethernet_box
  Bus Element In4 : Inport  Port=4  PortName=XGCS49 0 B201 _rtu_data_2_ethernet_box
  Bus Element In5 : Inport  Port=5  PortName=XGCS49 L B201 _rtu_data_2_ethernet_box
  Bus Element In6 : Inport  Port=6  PortName=XGCS 89 01201 _rtu_data_2_ethernet_box
  Bus Element Out1 : Outport  PortName=XGSZ 84 EIP _serial_data_ethernet

== system RFID/XGSZ 84 ETH  ==
  Bus Element In1 : Inport  PortName=M18_rtu_data_2_modbus_ box
  Bus Element In2 : Inport  Port=2  PortName=M30_rtu_data_2_modbus_box
  Bus Element In3 : Inport  Port=3  PortName=XGCS49 0 1201_rtu_data_2_modbus_box
  Bus Element In4 : Inport  Port=4  PortName=XGCS49 0 B201 _rtu_data_2_modbus_box
  Bus Element In5 : Inport  Port=5  PortName=XGCS49 L B201 _rtu_data_2_modbus_box
  Bus Element In6 : Inport  Port=6  PortName=XGCS 89 01201 _rtu_data_2_modbus_box
  Bus Element Out1 : Outport  PortName=XGSZ84 ETH _serial_data_Mobdus

== system RFID/XGSZ84 PNT  ==
  Bus Element In1 : Inport  PortName=""
  Bus Element In2 : Inport  Port=2  PortName=M30_rtu_data_2_profinet_box
  Bus Element In3 : Inport  Port=3  PortName=XGCS49 0 1201_rtu_data_2_profinet_box
  Bus Element In4 : Inport  Port=4  PortName=XGCS49 0 B201 _rtu_data_2_profinet_box
  Bus Element In5 : Inport  Port=5  PortName=XGCS49 L B201 _rtu_data_2_profinet_box
  Bus Element In6 : Inport  Port=6  PortName=XGCS 89 01201 _rtu_data_2_profinet_box
  Bus Element Out1 : Outport  PortName="XGSZ84 PNT  _serial_data_Profinet"

== system RFID/Control Module/CANJ Interface ==
  Bus Element In1 : Inport  PortName=CANJ_Sensor_fieldbus
  Bus Element Out1 : Outport  PortName=CANJ_Interface_Data

== system RFID/Control Module/Ethernet Interface ==
  Bus Element In1 : Inport  PortName=Ethernetip_Sensor_fieldbus
  Bus Element Out1 : Outport  PortName=Ethernet_Interface_Data

== system RFID/Control Module/IO Module ==
  Bus Element In1 : Inport  PortName=Descrete/Analog Input
  Bus Element Out1 : Outport  PortName=Descrete/Analog Data

== system RFID/Control Module/Modbus IIntereface ==
  Bus Element In1 : Inport  PortName=Modbus_Sensor_fieldbus
  Bus Element Out1 : Outport  PortName=Modbus_Intereface_Data

== system RFID/Control Module/PLC ==
  Bus Element In6 : Inport  PortName=Descrete/Analog Data
  Bus Element In5 : Inport  Port=2  PortName=CANJ_Interface_Data
  Bus Element In4 : Inport  Port=3  PortName=PLC_Programmation
  Bus Element In1 : Inport  Port=4  PortName=Profinet_Interface_Data
  Bus Element In2 : Inport  Port=5  PortName=Ethernet_Interface_Data
  Bus Element In3 : Inport  Port=6  PortName=Modbus_Intereface_Data
  Bus Element Out1 : Outport  PortName=Process_Parameters_HMI

== system RFID/Control Module/Profinet Interface ==
  Bus Element In1 : Inport  PortName=Profinet_Sensor_fieldbus
  Bus Element Out1 : Outport  PortName=Profinet_Interface_Data

== system RFID/RFID_CANJ/XGCS460B201 ==
  Bus Element Out1 : Outport  PortName=XGCS460B201_CANJ_Data

== system RFID/RFID_EthernetIP/XGCS 850C 201  ==
  Bus Element Out1 : Outport  PortName=XGCS 850C 201_Ethernetp_Data

== system RFID/RFID_IO_Link/M18 ==
  Bus Element Out1 : Outport  PortName=M18_IOLink_data

== system RFID/RFID_IO_Link/M30 ==
  Bus Element Out1 : Outport  PortName=M30_IOLink_data

== system RFID/RFID_IO_Link/XGCS 49 01201 ==
  Bus Element Out1 : Outport  PortName=XGCS 49 01201_IOLink_data

== system RFID/RFID_IO_Link/XGCS 89 01201 ==
  Bus Element Out1 : Outport  PortName=XGCS 89 01201_IOLimk_data

== system RFID/RFID_IO_Link1/M18 ==
  Bus Element Out1 : Outport  PortName=M18_IOLink_data

== system RFID/RFID_IO_Link1/M30 ==
  Bus Element Out1 : Outport  PortName=M30_IOLink_data

== system RFID/RFID_IO_Link1/XGCS 49 01201 ==
  Bus Element Out1 : Outport  PortName=XGCS 49 01201_IOLink_data

== system RFID/RFID_IO_Link1/XGCS 89 01201 ==
  Bus Element Out1 : Outport  PortName=XGCS 89 01201_IOLimk_data

== system RFID/RFID_Modbus/XGCS 850C 201 ==
  Bus Element Out1 : Outport  PortName=XGCS 850C 201_ModusTCp_Data

== system RFID/RFID_PNP/XGCS49 1 B201  ==
  Bus Element Out1 : Outport  PortName=XGCS49 1 B201_PNP_Data

== system RFID/RFID_Profinet/XGCS 850C 201  ==
  Bus Element Out1 : Outport  PortName=XGCS 850C 201_Profinet_Data

== system RFID/RFID_rtu/M18 ==
  Bus Element Out1 : Outport  PortName=M18_rtu_data

== system RFID/RFID_rtu/M30 ==
  Bus Element Out1 : Outport  PortName=M30_rtu_data

== system RFID/RFID_rtu/XGCS 89 01201  ==
  Bus Element Out1 : Outport  PortName=XGCS 89 01201 _rtu_data

== system RFID/RFID_rtu/XGCS49 0 1201  ==
  Bus Element Out1 : Outport  PortName=XGCS49 0 1201_rtu_data

== system RFID/RFID_rtu/XGCS49 0 B201  ==
  Bus Element Out1 : Outport  PortName=XGCS49 0 B201 _rtu_data

== system RFID/RFID_rtu/XGCS49 L B201  ==
  Bus Element Out1 : Outport  PortName=XGCS49 L B201 _rtu_data

== system RFID/RFID_rtu1/M18 ==
  Bus Element Out1 : Outport  PortName=M18_rtu_data

== system RFID/RFID_rtu1/M30 ==
  Bus Element Out1 : Outport  PortName=M30_rtu_data

== system RFID/RFID_rtu1/XGCS 89 01201  ==
  Bus Element Out1 : Outport  PortName=XGCS 89 01201 _rtu_data

== system RFID/RFID_rtu1/XGCS49 0 1201  ==
  Bus Element Out1 : Outport  PortName=XGCS49 0 1201_rtu_data

== system RFID/RFID_rtu1/XGCS49 0 B201  ==
  Bus Element Out1 : Outport  PortName=XGCS49 0 B201 _rtu_data

== system RFID/RFID_rtu1/XGCS49 L B201  ==
  Bus Element Out1 : Outport  PortName=XGCS49 L B201 _rtu_data

== system RFID/RFID_rtu2/M18 ==
  Bus Element Out1 : Outport  PortName=M18_rtu_data

== system RFID/RFID_rtu2/M30 ==
  Bus Element Out1 : Outport  PortName=M30_rtu_data

== system RFID/RFID_rtu2/XGCS 89 01201  ==
  Bus Element Out1 : Outport  PortName=XGCS 89 01201 _rtu_data

== system RFID/RFID_rtu2/XGCS49 0 1201  ==
  Bus Element Out1 : Outport  PortName=XGCS49 0 1201_rtu_data

== system RFID/RFID_rtu2/XGCS49 0 B201  ==
  Bus Element Out1 : Outport  PortName=XGCS49 0 B201 _rtu_data

== system RFID/RFID_rtu2/XGCS49 L B201  ==
  Bus Element Out1 : Outport  PortName=XGCS49 L B201 _rtu_data
